simulink model "Inertia_Calculate_65"  (Simulink 6.3)
settings: Solver=ode45  StartTime=0.0  StopTime=10.0  RelTol=1e-3
values from neighbouring files (symbols this model uses):
  mass = 54000    [Start.m]    (also in drl_simplified_dynamics.m)
  X = 1.06    [AircraftTrim.m]
settings Model: Creator=Administrator  LastModifiedBy=hp  StrictBusMsg=None
settings OptimizationCC: InitFltsAndDblsToZero=off
settings DebuggingCC: SignalResolutionControl=UseLocalSettings  MultiTaskDSMMsg=error
settings HardwareCC: TargetHWDeviceType=32-bit Generic

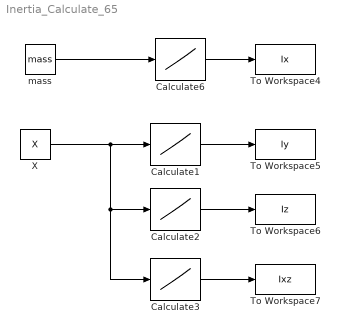
== system Inertia_Calculate_65 ==
  Calculate1 : Lookup  InputValues=[0.828 1.071 1.175]  OutputValues=[2317035.500 2218748.250 2288100.000]  OutDataType=fixdt(1, 16)
  Calculate2 : Lookup  InputValues=[0.828 1.071 1.175]  OutputValues=[4638430.000 4539179.000 4608704.000]  OutDataType=fixdt(1, 16)
  Calculate3 : Lookup  InputValues=[0.828 1.071 1.175]  OutputValues=[294446.500 285087.031 280069.906]  OutDataType=fixdt(1, 16)
  Calculate6 : Lookup  InputValues=[49000 54000 58000 61000 65000]  OutputValues=[1925039.000 2582750.000 2799186.500 2910520.500 2928538.250]  OutDataType=fixdt(1, 16)
  To Workspace4 : ToWorkspace  VariableName=Ix  SampleTime=-1  SaveFormat=Array
  To Workspace5 : ToWorkspace  VariableName=Iy  SampleTime=-1  SaveFormat=Array
  To Workspace6 : ToWorkspace  VariableName=Iz  SampleTime=-1  SaveFormat=Array
  To Workspace7 : ToWorkspace  VariableName=Ixz  SampleTime=-1  SaveFormat=Array
  X : Constant  Value=X  OutDataType=fixdt(1, 16)
  mass : Constant  Value=mass  OutDataType=fixdt(1, 16)
  wires:
  X/1 -> Calculate2/1, Calculate3/1, Calculate1/1
  Calculate1/1 -> To Workspace5/1
  Calculate2/1 -> To Workspace6/1
  Calculate3/1 -> To Workspace7/1
  Calculate6/1 -> To Workspace4/1
  mass/1 -> Calculate6/1
